simulink library "cic_library"  (Simulink 6.2)
libraries: xbsIndex_r3 x4, ddc_library x2
settings Model: LastModifiedBy=hchen05

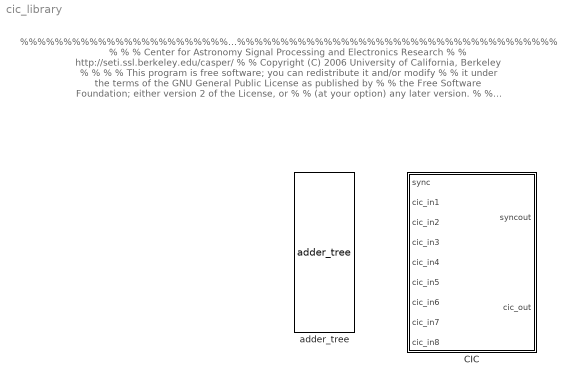
== system cic_library ==
  note: %%%%%%%%%%%%%%%%%%%%%%%%%%%%%%%%%%%%%%%%%%%%%%%%%%%%%%%%%%%%%%%%%%%%%%%%%%%%%%%
      | %                                                                             %
      | %   Center for Astronomy Signal Processing and Electronics Research           %
      | %   http://seti.ssl.berkeley.edu/casper/                                      %
      | %   Copyright (C) 2006 University of California, Berkeley                     %
      | %                                                                             %
      | %   This program is free software; you can redistribute it and/or modify      %
      | %   it under the terms of the GNU General Public License as published by      %
      | %   the Free Software Foundation; either version 2 of the License, or         %
      | %   (at your option) any later version.                                       %
      | %                                                                             %
      | %   This program is distributed in the hope that it will be useful,           %
      | %   but WITHOUT ANY WARRANTY; without even the implied warranty of            %
      | %   MERCHANTABILITY or FITNESS FOR A PARTICULAR PURPOSE.  See the             %
      | %   GNU General Public License for more details.                              %
      | %                                                                             %
      | %   You should have received a copy of the GNU General Public License along   %
      | %   with this program; if not, write to the Free Software Foundation, Inc.,   %
      | %   51 Franklin Street, Fifth Floor, Boston, MA 02110-1301 USA.               %
      | %                                                                             %
      | %%%%%%%%%%%%%%%%%%%%%%%%%%%%%%%%%%%%%%%%%%%%%%%%%%%%%%%%%%%%%%%%%%%%%%%%%%%%%%%
  CIC : Subsystem  Description="Cascaded integrator-comb filter.  Linear phase response."  mask(BEE2 CIC){inputs=8, input_bitwidth=8, input_binary_pt=7, D=1, R=1, stages=1, pipeline=off, add_latency=2, int_latency=1, comb_latency=1}
      mask prompts: input_bitwidth "Input bitwidth"; input_binary_pt "Input binary point"; D "Comb differential delay (D)"; R "Sample rate change (R) (2+ decimates; set to 1 for no decimation)"; stages "Number of stages"; add_latency "Adder latency"; int_latency "Integrator latency"; comb_latency "Comb latency"
      mask help: Cascaded integrator-comb filter. Linear phase response. Decimation only; no interpolation.
      mask init:
      | cic_mask;
      mask Help: eval('xlWeb([getenv(''MLIB_ROOT''), ''\astro_library\doc\cic_usage.html''])')
  adder_tree : ddc_library/adder_tree  num_inputs=inputs  latency=add_latency

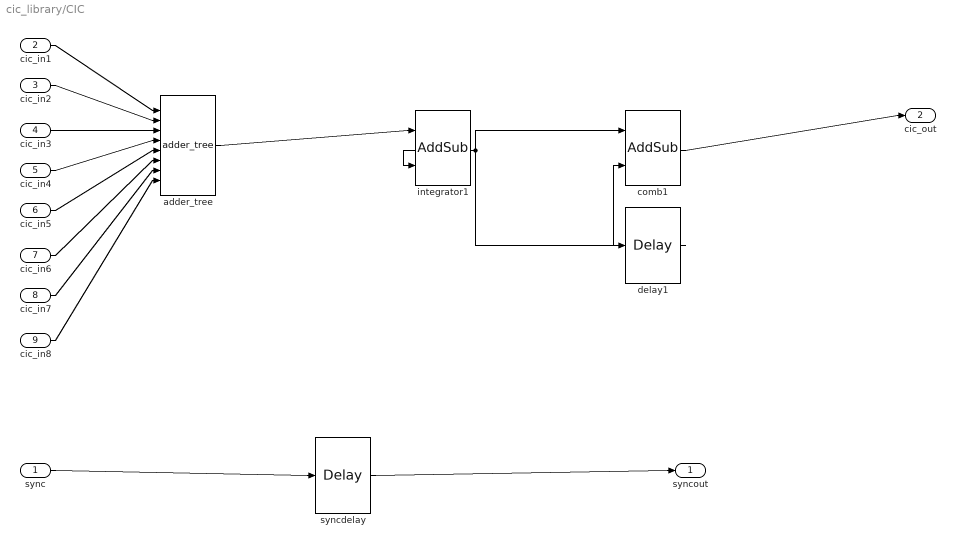
== system cic_library/CIC ==
  sync : Inport  Port=1  LatchInput=off
  cic_in1 : Inport  Port=2  LatchInput=off
  cic_in2 : Inport  Port=3  LatchInput=off
  cic_in3 : Inport  Port=4  LatchInput=off
  cic_in4 : Inport  Port=5  LatchInput=off
  cic_in5 : Inport  Port=6  LatchInput=off
  cic_in6 : Inport  Port=7  LatchInput=off
  cic_in7 : Inport  Port=8  LatchInput=off
  cic_in8 : Inport  Port=9  LatchInput=off
  adder_tree : ddc_library/adder_tree  num_inputs=inputs  latency=add_latency
  comb1 : xbsIndex_r3/AddSub  mode=Subtraction  precision=User Defined  arith_type="Signed  (2's comp)"  n_bits=ceil(input_bitwidth+log2(inputs)+stages*log2(R*D))  bin_pt=input_binary_pt  quantization=Truncate  overflow=Wrap  latency=comb_latency  explicit_period=on  period=1  use_carryin=off  use_carryout=off  en=off  dbl_ovrd=off  show_param=off  use_core=on  pipeline=on  use_rpm=on  gen_core=off
      settings: xl_area=[0, 0, 0, 0, 0, 0, 0]
  delay1 : xbsIndex_r3/Delay  latency=D  reg_retiming=off  explicit_period=off  period=1  en=off  accept_only_valid=off  init_zero=on  dbl_ovrd=off  show_param=off
      settings: xl_area=[0, 0, 0, 0, 0, 0, 0]
  integrator1 : xbsIndex_r3/AddSub  mode=Addition  precision=User Defined  arith_type="Signed  (2's comp)"  n_bits=ceil(input_bitwidth+log2(inputs)+stages*log2(R*D))  bin_pt=input_binary_pt  quantization=Truncate  overflow=Wrap  latency=int_latency  explicit_period=on  period=1  use_carryin=off  use_carryout=off  en=off  dbl_ovrd=off  show_param=off  use_core=on  pipeline=on  use_rpm=on  gen_core=off
      settings: xl_area=[0, 0, 0, 0, 0, 0, 0]
  syncdelay : xbsIndex_r3/Delay  latency=add_latency*log2(inputs)+stages*(int_latency+comb_latency+D+0)  reg_retiming=off  explicit_period=off  period=1  en=off  accept_only_valid=off  init_zero=on  dbl_ovrd=off  show_param=off
      settings: xl_area=[0, 0, 0, 0, 0, 0, 0]
  syncout : Outport
  cic_out : Outport  Port=2
  wires:
  sync/1 -> syncdelay/1
  syncdelay/1 -> syncout/1
  cic_in8/1 -> adder_tree/8
  cic_in7/1 -> adder_tree/7
  cic_in6/1 -> adder_tree/6
  cic_in5/1 -> adder_tree/5
  cic_in4/1 -> adder_tree/4
  cic_in3/1 -> adder_tree/3
  cic_in2/1 -> adder_tree/2
  cic_in1/1 -> adder_tree/1
  integrator1/1 -> comb1/1, delay1/1, integrator1/2
  adder_tree/1 -> integrator1/1
  comb1/1 -> cic_out/1
  delay1/1 -> comb1/2
